simulink model "malt_test_angle"  (R2022a)
settings: Solver=FixedStepAuto  StartTime=0.0  StopTime=50  FixedStep=framePeriod_s  RelTol=1e-3
undefined symbols (not defined in the file): Aircraft, DiscIntNeverNeededParam, framePeriod_s
libraries: simulink x29, slpidlib x8, simulink_extras x3
(part 2 of 2)

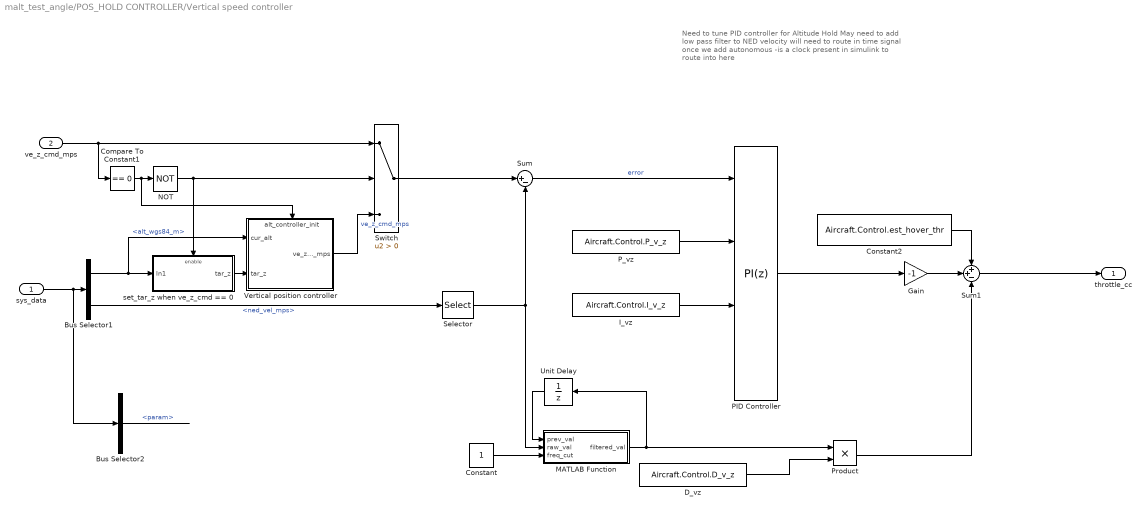
== system malt_test_angle/POS_HOLD CONTROLLER/Vertical speed controller ==
  note: Need to tune PID controller for Altitude Hold
      | May need to add low pass filter to NED velocity
      | will need to route in time signal once we add autonomous
      | -is a clock present in simulink to route into here
  sys_data : Inport
  ve_z_cmd_mps : Inport  Port=2
  Bus Selector1 : BusSelector  OutputSignals=Sensor Data.ext_gnss1.alt_wgs84_m,Sensor Data.ext_gnss1.ned_vel_mps
  Bus Selector2 : BusSelector  OutputSignals=Telemetry Data.param
  Compare To Constant1 : simulink/Logic and Bit Operations/Compare To Constant  relop===  const=0  OutDataTypeStr=boolean
  Constant : Constant
  Constant2 : Constant  Value=Aircraft.Control.est_hover_thr  OutDataTypeStr=single
  D_vz : Constant  Value=Aircraft.Control.D_v_z  OutDataTypeStr=single
  Gain : Gain  Gain=-1
  I_vz : Constant  Value=Aircraft.Control.I_v_z  OutDataTypeStr=single
  MATLAB Function : MATLAB Function  TreatAsAtomicUnit=on
  NOT : Logic  Operator=NOT  IconShape=distinctive  AllPortsSameDT=off  OutDataTypeStr=boolean
  PID Controller : slpidlib/PID Controller  Controller=PI  Form=Parallel  TimeDomain=Discrete-time  UseExternalTs=off  SampleTime=framePeriod_s  IntegratorMethod=Forward Euler  FilterMethod=Forward Euler  ControllerParametersSource=external  P=0  I=0  UseKiTs=off  D=0  N=100  UseFilter=off  TunerSelectOption=Frequency Response Based  InitialConditionSource=internal  InitialConditionForIntegrator=0  InitialConditionForFilter=0  DifferentiatorICPrevScaledInput=0  ExternalReset=either  TrackingMode=off  Kt=1  LimitOutput=on  SatLimitsSource=internal  UpperSaturationLimit=inf  LowerSaturationLimit=-inf  LinearizeAsGain=on  AntiWindupMode=clamping  Kb=1  POutMin=[]  POutMax=[]  IOutMin=[]  IOutMax=[]  DOutMin=[]  DOutMax=[]  NOutMin=[]  NOutMax=[]  SumOutMin=[]  SumOutMax=[]  SaturationOutMin=[]  SaturationOutMax=[]  PParamMin=[]  PParamMax=[]  IParamMin=[]  IParamMax=[]  DParamMin=[]  DParamMax=[]  NParamMin=[]  NParamMax=[]  KbParamMin=[]  KbParamMax=[]  KtParamMin=[]  KtParamMax=[]  KbOutMin=[]  KbOutMax=[]  KtOutMin=[]  KtOutMax=[]  IntegratorOutMin=[]  IntegratorOutMax=[]  FilterOutMin=[]  FilterOutMax=[]  SumI1OutMin=[]  SumI1OutMax=[]  SumI2OutMin=[]  SumI2OutMax=[]  SumI3OutMin=[]  SumI3OutMax=[]  SumI4OutMin=[]  SumI4OutMax=[]  SumDOutMin=[]  SumDOutMax=[]  DifferentiatorOutMin=[]  DifferentiatorOutMax=[]  FilterDiffOutCoefMin=[]  FilterDiffOutCoefMax=[]  ReciprocalOutMin=[]  ReciprocalOutMax=[]  SumDenOutMin=[]  SumDenOutMax=[]  SumNumOutMin=[]  SumNumOutMax=[]  DivideOutMin=[]  DivideOutMax=[]  UdiffTsProdOutMin=[]  UdiffTsProdOutMax=[]  NTsProdOutMin=[]  NTsProdOutMax=[]  UintegralTsProdOutMin=[]  UintegralTsProdOutMax=[]  UngainTsProdOutMin=[]  UngainTsProdOutMax=[]  IntegratorContinuousStateAttributes=''  IntegratorStateMustResolveToSignalObject=off  IntegratorRTWStateStorageClass=Auto  FilterContinuousStateAttributes=''  FilterStateMustResolveToSignalObject=off  FilterRTWStateStorageClass=Auto  ParallelPVariant=ExternalParameters  IdealPVariant=Disabled  IVariant=ExternalParameters  DVariant=Disabled  IntegratorVariant=Discrete  SatVariant=Enabled  AWVariant=DiscClampingParallel  PCopyVariant=Disabled  TRVariant=Disabled  FdbkBlocksVariant=Forward  IdealPFdbkVariant=Disabled  SatFdbkVariant=Disabled  DerivativeFilterVariant=Disabled  NVariant=Disabled  NCopyVariant=Disabled_SignalSpec  FilterICVariant=Disabled  IntegratorICVariant=InternalICs  ExternalResetVariant=ExternalReset  TRSumVariant=Passthrough  SumFdbkVariant=Disabled  SumVariant=Sum_PI  TsampFilterVariant=InternalTs  TsampNgainVariant=Passthrough  TsampIntegralVariant=Passthrough  ExternalSaturationOutDataTypeStr=Inherit: Same as second input  aMode=0
  P_vz : Constant  Value=Aircraft.Control.P_v_z  OutDataTypeStr=single
  Product : Product
  Selector : Selector  InputPortWidth=3  IndexOptions=Index vector (dialog)  Indices=[3]  OutputSizes=1
  Sum : Sum  Inputs=|+-
  Sum1 : Sum  Inputs=++-
  Switch : Switch  Criteria=u2 > Threshold  SaturateOnIntegerOverflow=off  InputSameDT=off
  Unit Delay : UnitDelay  SampleTime=-1  HasFrameUpgradeWarning=on
  Vertical position controller : Subsystem
      settings: PortSchema="{\"entries\":[{\"content\":{\"sides\":[{\"content\":{\"connectorIds\":[\"In1\",\"In2\"]},\"type\":\"ConnectorPlacement.EquallySpacedRectSide\",\"uuid\":\"4db66816-7259-4f9c-97dc-3e2ef8fc1f9a\"},{\"content\":{\"connectorIds\":[\"Out1\"],\"side\":\"RIGHT\"},\"type\":\"ConnectorPlacement.EquallySpacedRectSide\",\"uuid\":\"8b35fa77-d974-4b31-bf6a-1bec360e39d1\"},{\"content\":{\"connectorIds\":[\"In3\"],\"side\":\"TOP\"},\"type\":\"ConnectorPlacement.EquallySpacedRectSide\",\"uuid\":\"3ae99705-2896-4d33-823c-501dd4ab52dc\"}]},\"type\":\"ConnectorPlacement.EquallySpacedConnector\",\"uuid\":\"6b05b274-635e-41e6-a26b-037c1baff98b\"}],\"packageUris\":[\"http://schema.mathworks.com/mf0/Connector/R2020b\"],\"version\":\"1.0\"}"
  set_tar_z when ve_z_cmd == 0 : Subsystem  TreatAsAtomicUnit=on
  throttle_cc : Outport
  wires:
  Sum/1 -> PID Controller/1  "error"
  I_vz/1 -> PID Controller/3
  P_vz/1 -> PID Controller/2
  PID Controller/1 -> Gain/1
  Bus Selector1/2 -> Selector/1  "<ned_vel_mps>"
  sys_data/1 -> Bus Selector2/1, Bus Selector1/1
  Sum1/1 -> throttle_cc/1
  Bus Selector2/1 -> ?  "<param>"
  Unit Delay/1 -> MATLAB Function/1(prev_val)
  MATLAB Function/1(filtered_val) -> Product/1, Unit Delay/1
  Selector/1 -> Sum/2, MATLAB Function/2(raw_val)
  Constant/1 -> MATLAB Function/3(freq_cut)
  D_vz/1 -> Product/2
  Constant2/1 -> Sum1/1
  Gain/1 -> Sum1/2
  Product/1 -> Sum1/3
  ve_z_cmd_mps/1 -> Compare To Constant1/1, Switch/1
  Compare To Constant1/1 -> Vertical position controller/3(alt_controller_init), NOT/1
  Bus Selector1/1 -> Vertical position controller/1(cur_alt), set_tar_z when ve_z_cmd == 0/1(In1)  "<alt_wgs84_m>"
  NOT/1 -> Switch/2, set_tar_z when ve_z_cmd == 0/Enable
  Switch/1 -> Sum/1
  set_tar_z when ve_z_cmd == 0/1(tar_z) -> Vertical position controller/2(tar_z)
  Vertical position controller/1(ve_z_cmd_mps) -> Switch/3  "ve_z_cmd_mps"

== system malt_test_angle/Stab_input_conversion/remap from min_spin to max ==
  raw_in : Inport
  Constant4 : Constant  Value=0  OutDataTypeStr=single
  Constant5 : Constant  Value=Aircraft.Control.motor_spin_min  OutDataTypeStr=single
  Constant6 : Constant  OutDataTypeStr=single
  Constant7 : Constant  OutDataTypeStr=single
  remap1 : MATLAB Function  TreatAsAtomicUnit=on
  norm_out : Outport
  wires:
  Constant6/1 -> remap1/5(out_max)
  Constant5/1 -> remap1/4(out_min)
  remap1/1(norm_out) -> norm_out/1
  Constant4/1 -> remap1/2(in_min)
  Constant7/1 -> remap1/3(in_max)
  raw_in/1 -> remap1/1(raw_in)

== system malt_test_angle/Stab_input_conversion1/Throttle Mapper ==
  Throttle : Inport
  Compare To Constant : simulink/Logic and Bit Operations/Compare To Constant  relop=<  const=0  OutDataTypeStr=boolean
  Compare To Constant1 : simulink/Logic and Bit Operations/Compare To Constant  relop=>=  const=0  OutDataTypeStr=boolean
  Constant : Constant  Value=Aircraft.Control.v_z_down_max  OutDataTypeStr=single
  Constant1 : Constant  Value=Aircraft.Control.v_z_up_max  OutDataTypeStr=single
  Double : Constant  Value=2  OutDataTypeStr=single
  Gain : Gain  Gain=-1
  Normalize at Zero : Constant  Value=0.5  OutDataTypeStr=single
  Product : Product  Inputs=3
  Product1 : Product  Inputs=3
  Sum : Sum  Inputs=|+-
  Sum1 : Sum
  v_z_cmd (-1 to 1) : Product
  Relative Velocity : Outport
  wires:
  Throttle/1 -> Sum/1
  Normalize at Zero/1 -> Sum/2
  Double/1 -> v_z_cmd (-1 to 1)/2
  Sum/1 -> v_z_cmd (-1 to 1)/1
  Sum1/1 -> Gain/1
  v_z_cmd (-1 to 1)/1 -> Product1/2, Compare To Constant1/1, Compare To Constant/1, Product/3
  Constant1/1 -> Product1/3
  Compare To Constant1/1 -> Product1/1
  Product/1 -> Sum1/1
  Product1/1 -> Sum1/2
  Constant/1 -> Product/1
  Compare To Constant/1 -> Product/2
  Gain/1 -> Relative Velocity/1

== system malt_test_angle/Stab_input_conversion1/pitch_norm_deadband ==
  raw_sbus_in : Inport
  deadband : Inport  Port=2
  Constant : Constant  Value=0  OutDataTypeStr=single
  Constant1 : Constant  Value=0  OutDataTypeStr=single
  Constant2 : Constant  OutDataTypeStr=single
  Constant3 : Constant  OutDataTypeStr=single
  remap_with_deadband : MATLAB Function  TreatAsAtomicUnit=on
  normalized_out : Outport
  wires:
  deadband/1 -> remap_with_deadband/6(deadband)
  Constant2/1 -> remap_with_deadband/5(out_max)
  Constant1/1 -> remap_with_deadband/4(out_min)
  Constant3/1 -> remap_with_deadband/3(in_max)
  Constant/1 -> remap_with_deadband/2(in_min)
  remap_with_deadband/1(norm_out) -> normalized_out/1
  raw_sbus_in/1 -> remap_with_deadband/1(raw_in)

== system malt_test_angle/cmd to raw pwm1/motor_PWM_denormalize ==
  normalized_input : Inport
  Constant : Constant  Value=0  OutDataTypeStr=single
  Constant1 : Constant  Value=1100  OutDataTypeStr=single
  Constant2 : Constant  Value=1950  OutDataTypeStr=single
  Constant3 : Constant  OutDataTypeStr=single
  remap : MATLAB Function  TreatAsAtomicUnit=on
  raw_output : Outport
  wires:
  Constant2/1 -> remap/5(out_max)
  Constant1/1 -> remap/4(out_min)
  Constant3/1 -> remap/3(in_max)
  Constant/1 -> remap/2(in_min)
  remap/1(raw_out) -> raw_output/1
  normalized_input/1 -> remap/1(norm_in)

== system malt_test_angle/command selection/e_stop_norm ==
  raw_sbus_in : Inport
  Constant : Constant  Value=172  OutDataTypeStr=single
  Constant1 : Constant  Value=-1  OutDataTypeStr=single
  Constant2 : Constant  OutDataTypeStr=single
  Constant3 : Constant  Value=1811  OutDataTypeStr=single
  remap : MATLAB Function  TreatAsAtomicUnit=on
  normalized_out : Outport
  wires:
  Constant2/1 -> remap/5(out_max)
  Constant1/1 -> remap/4(out_min)
  Constant3/1 -> remap/3(in_max)
  Constant/1 -> remap/2(in_min)
  remap/1(norm_out) -> normalized_out/1
  raw_sbus_in/1 -> remap/1(raw_in)

== system malt_test_angle/command selection/mode_norm ==
  raw_sbus_in : Inport
  Constant : Constant  Value=172  OutDataTypeStr=single
  Constant1 : Constant  Value=0  OutDataTypeStr=single
  Constant2 : Constant  Value=2  OutDataTypeStr=single
  Constant3 : Constant  Value=1811  OutDataTypeStr=single
  remap : MATLAB Function  TreatAsAtomicUnit=on
  normalized_out : Outport
  wires:
  raw_sbus_in/1 -> remap/1(raw_in)
  remap/1(norm_out) -> normalized_out/1
  Constant/1 -> remap/2(in_min)
  Constant3/1 -> remap/3(in_max)
  Constant1/1 -> remap/4(out_min)
  Constant2/1 -> remap/5(out_max)

== system malt_test_angle/command selection/pitch_norm_deadband ==
  raw_sbus_in : Inport
  deadband : Inport  Port=2
  Constant : Constant  Value=172  OutDataTypeStr=single
  Constant1 : Constant  Value=-1  OutDataTypeStr=single
  Constant2 : Constant  OutDataTypeStr=single
  Constant3 : Constant  Value=1811  OutDataTypeStr=single
  remap_with_deadband : MATLAB Function  TreatAsAtomicUnit=on
  normalized_out : Outport
  wires:
  deadband/1 -> remap_with_deadband/6(deadband)
  Constant2/1 -> remap_with_deadband/5(out_max)
  Constant1/1 -> remap_with_deadband/4(out_min)
  Constant3/1 -> remap_with_deadband/3(in_max)
  Constant/1 -> remap_with_deadband/2(in_min)
  remap_with_deadband/1(norm_out) -> normalized_out/1
  raw_sbus_in/1 -> remap_with_deadband/1(raw_in)

== system malt_test_angle/command selection/roll_norm_deadband ==
  raw_sbus_in : Inport
  deadband : Inport  Port=2
  Constant : Constant  Value=172  OutDataTypeStr=single
  Constant1 : Constant  Value=-1  OutDataTypeStr=single
  Constant2 : Constant  OutDataTypeStr=single
  Constant3 : Constant  Value=1811  OutDataTypeStr=single
  remap_with_deadband : MATLAB Function  TreatAsAtomicUnit=on
  normalized_out : Outport
  wires:
  deadband/1 -> remap_with_deadband/6(deadband)
  Constant2/1 -> remap_with_deadband/5(out_max)
  Constant1/1 -> remap_with_deadband/4(out_min)
  Constant3/1 -> remap_with_deadband/3(in_max)
  Constant/1 -> remap_with_deadband/2(in_min)
  remap_with_deadband/1(norm_out) -> normalized_out/1
  raw_sbus_in/1 -> remap_with_deadband/1(raw_in)

== system malt_test_angle/command selection/throttle_norm ==
  raw_sbus_in : Inport
  Constant : Constant  Value=172  OutDataTypeStr=single
  Constant1 : Constant  Value=0  OutDataTypeStr=single
  Constant2 : Constant  OutDataTypeStr=single
  Constant3 : Constant  Value=1811  OutDataTypeStr=single
  remap : MATLAB Function  TreatAsAtomicUnit=on
  normalized_out : Outport
  wires:
  raw_sbus_in/1 -> remap/1(raw_in)
  remap/1(norm_out) -> normalized_out/1
  Constant/1 -> remap/2(in_min)
  Constant3/1 -> remap/3(in_max)
  Constant1/1 -> remap/4(out_min)
  Constant2/1 -> remap/5(out_max)

== system malt_test_angle/command selection/yaw_norm_deadband ==
  raw_sbus_in : Inport
  deadband : Inport  Port=2
  Constant : Constant  Value=172  OutDataTypeStr=single
  Constant1 : Constant  Value=-1  OutDataTypeStr=single
  Constant2 : Constant  OutDataTypeStr=single
  Constant3 : Constant  Value=1811  OutDataTypeStr=single
  remap_with_deadband : MATLAB Function  TreatAsAtomicUnit=on
  normalized_out : Outport
  wires:
  raw_sbus_in/1 -> remap_with_deadband/1(raw_in)
  remap_with_deadband/1(norm_out) -> normalized_out/1
  Constant/1 -> remap_with_deadband/2(in_min)
  Constant3/1 -> remap_with_deadband/3(in_max)
  Constant1/1 -> remap_with_deadband/4(out_min)
  Constant2/1 -> remap_with_deadband/5(out_max)
  deadband/1 -> remap_with_deadband/6(deadband)

== system malt_test_angle/determine arm and mode selection/Failsafe_management ==
  note: - radio failsafe
  In Bus Element1 : Inport  PortName=failsafe  Element=failsafe
  manual_mode : Inport  Port=2
  motor_state : Inport  Port=3
  NOT : Logic  Operator=NOT  IconShape=distinctive  AllPortsSameDT=off  OutDataTypeStr=boolean
  Radio failsafe : Subsystem
  radio_failsafe_enabled : Outport
  wires:
  Radio failsafe/1(radio_failsafe_enabled) -> radio_failsafe_enabled/1
  manual_mode/1 -> [manual_mode], Radio failsafe/2(manual_mode)
  motor_state/1 -> Radio failsafe/3(motor_state)
  In Bus Element1/1 -> NOT/1
  NOT/1 -> Radio failsafe/1(failsafe)

== system malt_test_angle/determine arm and mode selection/Subsystem ==
  <e_stop> : Inport
  Abs1 : Abs  SaturateOnIntegerOverflow=off
  Compare To Constant : simulink/Logic and Bit Operations/Compare To Constant  relop=>=  const=0.98  OutDataTypeStr=boolean
  e_stop counter : Subsystem
  e_stop_filtered : Outport
  wires:
  Compare To Constant/1 -> e_stop counter/Enable
  Abs1/1 -> Compare To Constant/1
  <e_stop>/1 -> e_stop counter/1(motor_e_stop_raw), Abs1/1
  e_stop counter/1(e_stop_filtered) -> e_stop_filtered/1

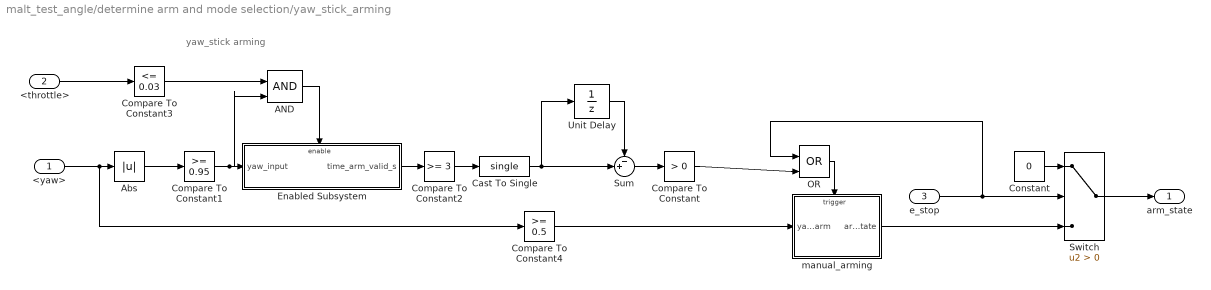
== system malt_test_angle/determine arm and mode selection/yaw_stick_arming ==
  note: yaw_stick arming
  <yaw> : Inport
  <throttle> : Inport  Port=2
  e_stop : Inport  Port=3
  AND : Logic  IconShape=distinctive  AllPortsSameDT=off  OutDataTypeStr=boolean
  Abs : Abs  SaturateOnIntegerOverflow=off
  Cast To Single : DataTypeConversion  OutDataTypeStr=single  SaturateOnIntegerOverflow=off  RndMeth=Floor
  Compare To Constant : simulink/Logic and Bit Operations/Compare To Constant  relop=>  const=0  OutDataTypeStr=boolean
  Compare To Constant1 : simulink/Logic and Bit Operations/Compare To Constant  relop=>=  const=0.95  OutDataTypeStr=boolean
  Compare To Constant2 : simulink/Logic and Bit Operations/Compare To Constant  relop=>=  const=3  OutDataTypeStr=boolean
  Compare To Constant3 : simulink/Logic and Bit Operations/Compare To Constant  relop=<=  const=0.03  OutDataTypeStr=boolean
  Compare To Constant4 : simulink/Logic and Bit Operations/Compare To Constant  relop=>=  const=0.5  OutDataTypeStr=boolean
  Constant : Constant  Value=0  OutDataTypeStr=boolean  LockScale=on
  Enabled Subsystem : Subsystem  TreatAsAtomicUnit=on
  OR : Logic  Operator=OR  IconShape=distinctive  AllPortsSameDT=off  OutDataTypeStr=boolean
  Sum : Sum  Inputs=-+|
  Switch : Switch  Criteria=u2 > Threshold  SaturateOnIntegerOverflow=off  InputSameDT=off
  Unit Delay : UnitDelay  SampleTime=-1  HasFrameUpgradeWarning=on
  manual_arming : Subsystem
  arm_state : Outport
  wires:
  Enabled Subsystem/1(time_arm_valid_s) -> Compare To Constant2/1
  Abs/1 -> Compare To Constant1/1
  Compare To Constant1/1 -> AND/2, Enabled Subsystem/1(yaw_input)
  Compare To Constant4/1 -> manual_arming/1(yaw_arm)
  AND/1 -> Enabled Subsystem/Enable
  <yaw>/1 -> Compare To Constant4/1, Abs/1
  <throttle>/1 -> Compare To Constant3/1
  Compare To Constant3/1 -> AND/1
  Constant/1 -> Switch/1
  manual_arming/1(arm_state) -> Switch/3
  Switch/1 -> arm_state/1
  e_stop/1 -> OR/1, Switch/2
  OR/1 -> manual_arming/Trigger
  Compare To Constant2/1 -> Cast To Single/1
  Sum/1 -> Compare To Constant/1
  Unit Delay/1 -> Sum/1
  Cast To Single/1 -> Unit Delay/1, Sum/2
  Compare To Constant/1 -> OR/2

== system malt_test_angle/ANGLE CONTROLLER1/Pitch Controller/Pitch_D_DLPF ==
  raw_val : Inport
  freq_cut : Inport  Port=2
  MATLAB Function : MATLAB Function  TreatAsAtomicUnit=on
  Unit Delay : UnitDelay  SampleTime=-1  HasFrameUpgradeWarning=on
  filtered_val : Outport
  wires:
  MATLAB Function/1(filtered_val) -> filtered_val/1, Unit Delay/1
  raw_val/1 -> MATLAB Function/2(raw_val)
  Unit Delay/1 -> MATLAB Function/1(prev_val)
  freq_cut/1 -> MATLAB Function/3(freq_cut)

== system malt_test_angle/ANGLE CONTROLLER1/Roll Controller/roll_D_DLPF ==
  raw_val : Inport
  freq_cut : Inport  Port=2
  MATLAB Function : MATLAB Function  TreatAsAtomicUnit=on
  Unit Delay : UnitDelay  SampleTime=-1  HasFrameUpgradeWarning=on
  filtered_val : Outport
  wires:
  freq_cut/1 -> MATLAB Function/3(freq_cut)
  MATLAB Function/1(filtered_val) -> filtered_val/1, Unit Delay/1
  Unit Delay/1 -> MATLAB Function/1(prev_val)
  raw_val/1 -> MATLAB Function/2(raw_val)

== system malt_test_angle/ANGLE CONTROLLER1/Yaw Rate Controller/heading_error ==
  heading_cmd_rad : Inport
  heading_rad : Inport  Port=2
  Abs : Abs  SaturateOnIntegerOverflow=off
  Compare To Constant : simulink/Logic and Bit Operations/Compare To Constant  relop=>  const=pi  OutDataTypeStr=boolean
  Constant : Constant  Value=2*pi  OutDataTypeStr=single
  Product : Product
  Sign : Signum
  Subtract : Sum  Inputs=+-
  Subtract1 : Sum  Inputs=+-
  Switch : Switch  Criteria=u2 > Threshold  SaturateOnIntegerOverflow=off  InputSameDT=off
  heading_error_rad : Outport
  wires:
  heading_cmd_rad/1 -> Subtract/1
  heading_rad/1 -> Subtract/2
  Subtract/1 -> Abs/1, Switch/3, Subtract1/1, Sign/1
  Compare To Constant/1 -> Switch/2
  Subtract1/1 -> Switch/1
  Switch/1 -> heading_error_rad/1
  Abs/1 -> Compare To Constant/1
  Sign/1 -> Product/1
  Product/1 -> Subtract1/2
  Constant/1 -> Product/2

== system malt_test_angle/ANGLE CONTROLLER1/Yaw Rate Controller/set_tar_heading when heading_rate_cmd == 0 ==
  heading_rad : Inport
  Enable : EnablePort
  target_heading_rad : Outport
  wires:
  heading_rad/1 -> target_heading_rad/1

== system malt_test_angle/ANGLE CONTROLLER1/Yaw Rate Controller/yaw_D_DLPF ==
  raw_val : Inport
  freq_cut : Inport  Port=2
  MATLAB Function : MATLAB Function  TreatAsAtomicUnit=on
  Unit Delay : UnitDelay  SampleTime=-1  HasFrameUpgradeWarning=on
  filtered_val : Outport
  wires:
  Unit Delay/1 -> MATLAB Function/1(prev_val)
  raw_val/1 -> MATLAB Function/2(raw_val)
  MATLAB Function/1(filtered_val) -> filtered_val/1, Unit Delay/1
  freq_cut/1 -> MATLAB Function/3(freq_cut)

== system malt_test_angle/POS_HOLD CONTROLLER/Horizontal speed controller/2D rotation from NED_xy to body_xy ==
  <heading_rad> : Inport
  Cos : Trigonometry  Operator=cos  OutputSignalType=real
  Gain : Gain  Gain=-1
  Mux : Mux
  Reshape : Reshape  OutputDimensionality=Customize  OutputDimensions=[2,2]
  Sin : Trigonometry  OutputSignalType=real
  2D_rot : Outport
  wires:
  <heading_rad>/1 -> Sin/1, Cos/1
  Mux/1 -> Reshape/1
  Sin/1 -> Mux/3, Gain/1
  Cos/1 -> Mux/1, Mux/4
  Reshape/1 -> 2D_rot/1
  Gain/1 -> Mux/2

== system malt_test_angle/POS_HOLD CONTROLLER/Horizontal speed controller/Subsystem ==
  vb_x cmd : Inport
  vb_x : Inport  Port=2
  pos_hold_p : Inport  Port=3
  pos_hold_I : Inport  Port=4
  pos_hold_D : Inport  Port=5
  pos_hold_init : Inport  Port=6
  Gain : Gain  Gain=-1
  Gain Selector : Subsystem  Commented=through
  Gain Selector1 : Subsystem  Commented=through
  Gain Selector2 : Subsystem  Commented=through
  Pitch angle controller : slpidlib/PID Controller  Controller=PID  Form=Parallel  TimeDomain=Discrete-time  UseExternalTs=off  SampleTime=framePeriod_s  IntegratorMethod=Forward Euler  FilterMethod=Forward Euler  ControllerParametersSource=external  P=0.335  I=0.005  UseKiTs=off  D=0  N=100  UseFilter=off  TunerSelectOption=Transfer Function Based (PID Tuner App)  InitialConditionSource=internal  InitialConditionForIntegrator=0  InitialConditionForFilter=0  DifferentiatorICPrevScaledInput=0  ExternalReset=rising  TrackingMode=off  Kt=1  LimitOutput=on  SatLimitsSource=internal  UpperSaturationLimit=inf  LowerSaturationLimit=-inf  LinearizeAsGain=off  AntiWindupMode=clamping  Kb=1  POutMin=[]  POutMax=[]  IOutMin=[]  IOutMax=[]  DOutMin=[]  DOutMax=[]  NOutMin=[]  NOutMax=[]  SumOutMin=[]  SumOutMax=[]  SaturationOutMin=[]  SaturationOutMax=[]  PParamMin=[]  PParamMax=[]  IParamMin=[]  IParamMax=[]  DParamMin=[]  DParamMax=[]  NParamMin=[]  NParamMax=[]  KbParamMin=[]  KbParamMax=[]  KtParamMin=[]  KtParamMax=[]  KbOutMin=[]  KbOutMax=[]  KtOutMin=[]  KtOutMax=[]  IntegratorOutMin=[]  IntegratorOutMax=[]  FilterOutMin=[]  FilterOutMax=[]  SumI1OutMin=[]  SumI1OutMax=[]  SumI2OutMin=[]  SumI2OutMax=[]  SumI3OutMin=[]  SumI3OutMax=[]  SumI4OutMin=[]  SumI4OutMax=[]  SumDOutMin=[]  SumDOutMax=[]  DifferentiatorOutMin=[]  DifferentiatorOutMax=[]  FilterDiffOutCoefMin=[]  FilterDiffOutCoefMax=[]  ReciprocalOutMin=[]  ReciprocalOutMax=[]  SumDenOutMin=[]  SumDenOutMax=[]  SumNumOutMin=[]  SumNumOutMax=[]  DivideOutMin=[]  DivideOutMax=[]  UdiffTsProdOutMin=[]  UdiffTsProdOutMax=[]  NTsProdOutMin=[]  NTsProdOutMax=[]  UintegralTsProdOutMin=[]  UintegralTsProdOutMax=[]  UngainTsProdOutMin=[]  UngainTsProdOutMax=[]  IntegratorContinuousStateAttributes=''  IntegratorStateMustResolveToSignalObject=off  IntegratorRTWStateStorageClass=Auto  FilterContinuousStateAttributes=''  FilterStateMustResolveToSignalObject=off  FilterRTWStateStorageClass=Auto  ParallelPVariant=ExternalParameters  IdealPVariant=Disabled  IVariant=ExternalParameters  DVariant=ExternalParameters  IntegratorVariant=Discrete  SatVariant=Enabled  AWVariant=DiscClampingParallel  PCopyVariant=Disabled  TRVariant=Disabled  FdbkBlocksVariant=Forward  IdealPFdbkVariant=Disabled  SatFdbkVariant=Disabled  DerivativeFilterVariant=Differentiator  NVariant=Passthrough  NCopyVariant=Disabled_SignalSpec  FilterICVariant=InternalICsDifferentiator  IntegratorICVariant=InternalICs  ExternalResetVariant=ExternalReset  TRSumVariant=Passthrough  SumFdbkVariant=Disabled  SumVariant=Sum_PID  TsampFilterVariant=InternalTs  TsampNgainVariant=Passthrough  TsampIntegralVariant=Passthrough  ExternalSaturationOutDataTypeStr=Inherit: Same as second input  aMode=0
  Saturation : Saturate  UpperLimit=Aircraft.Control.pitch_angle_lim  LowerLimit=-Aircraft.Control.pitch_angle_lim  LinearizeAsGain=off
  Sum : Sum  Inputs=|+-
  pitch_cmd_rad : Outport
  wires:
  vb_x/1 -> Sum/2
  Sum/1 -> Pitch angle controller/1
  vb_x cmd/1 -> Sum/1
  Saturation/1 -> Gain/1
  Pitch angle controller/1 -> Saturation/1
  Gain/1 -> pitch_cmd_rad/1
  pos_hold_I/1 -> Gain Selector1/1(param)
  pos_hold_p/1 -> Gain Selector/1(param)
  Gain Selector/1(gain) -> Pitch angle controller/2
  Gain Selector1/1(gain) -> Pitch angle controller/3  "I_gain"
  Gain Selector2/1(gain) -> Pitch angle controller/4  "I_gain"
  pos_hold_D/1 -> Gain Selector2/1(param)
  pos_hold_init/1 -> Pitch angle controller/5

== system malt_test_angle/POS_HOLD CONTROLLER/Horizontal speed controller/Subsystem1 ==
  vb_y : Inport
  vb_y cmd : Inport  Port=2
  pos_hold_p : Inport  Port=3
  pos_hold_I : Inport  Port=4
  pos_hold_D : Inport  Port=5
  pos_hold_init : Inport  Port=6
  Gain Selector : Subsystem  Commented=through
  Gain Selector1 : Subsystem  Commented=through
  Gain Selector2 : Subsystem  Commented=through
  Roll angle controller : slpidlib/PID Controller  Controller=PID  Form=Parallel  TimeDomain=Discrete-time  UseExternalTs=off  SampleTime=framePeriod_s  IntegratorMethod=Forward Euler  FilterMethod=Forward Euler  ControllerParametersSource=external  P=0.335  I=0.005  UseKiTs=off  D=0  N=100  UseFilter=off  TunerSelectOption=Transfer Function Based (PID Tuner App)  InitialConditionSource=internal  InitialConditionForIntegrator=0  InitialConditionForFilter=0  DifferentiatorICPrevScaledInput=0  ExternalReset=rising  TrackingMode=off  Kt=1  LimitOutput=on  SatLimitsSource=internal  UpperSaturationLimit=inf  LowerSaturationLimit=-inf  LinearizeAsGain=off  AntiWindupMode=clamping  Kb=1  POutMin=[]  POutMax=[]  IOutMin=[]  IOutMax=[]  DOutMin=[]  DOutMax=[]  NOutMin=[]  NOutMax=[]  SumOutMin=[]  SumOutMax=[]  SaturationOutMin=[]  SaturationOutMax=[]  PParamMin=[]  PParamMax=[]  IParamMin=[]  IParamMax=[]  DParamMin=[]  DParamMax=[]  NParamMin=[]  NParamMax=[]  KbParamMin=[]  KbParamMax=[]  KtParamMin=[]  KtParamMax=[]  KbOutMin=[]  KbOutMax=[]  KtOutMin=[]  KtOutMax=[]  IntegratorOutMin=[]  IntegratorOutMax=[]  FilterOutMin=[]  FilterOutMax=[]  SumI1OutMin=[]  SumI1OutMax=[]  SumI2OutMin=[]  SumI2OutMax=[]  SumI3OutMin=[]  SumI3OutMax=[]  SumI4OutMin=[]  SumI4OutMax=[]  SumDOutMin=[]  SumDOutMax=[]  DifferentiatorOutMin=[]  DifferentiatorOutMax=[]  FilterDiffOutCoefMin=[]  FilterDiffOutCoefMax=[]  ReciprocalOutMin=[]  ReciprocalOutMax=[]  SumDenOutMin=[]  SumDenOutMax=[]  SumNumOutMin=[]  SumNumOutMax=[]  DivideOutMin=[]  DivideOutMax=[]  UdiffTsProdOutMin=[]  UdiffTsProdOutMax=[]  NTsProdOutMin=[]  NTsProdOutMax=[]  UintegralTsProdOutMin=[]  UintegralTsProdOutMax=[]  UngainTsProdOutMin=[]  UngainTsProdOutMax=[]  IntegratorContinuousStateAttributes=''  IntegratorStateMustResolveToSignalObject=off  IntegratorRTWStateStorageClass=Auto  FilterContinuousStateAttributes=''  FilterStateMustResolveToSignalObject=off  FilterRTWStateStorageClass=Auto  ParallelPVariant=ExternalParameters  IdealPVariant=Disabled  IVariant=ExternalParameters  DVariant=ExternalParameters  IntegratorVariant=Discrete  SatVariant=Enabled  AWVariant=DiscClampingParallel  PCopyVariant=Disabled  TRVariant=Disabled  FdbkBlocksVariant=Forward  IdealPFdbkVariant=Disabled  SatFdbkVariant=Disabled  DerivativeFilterVariant=Differentiator  NVariant=Passthrough  NCopyVariant=Disabled_SignalSpec  FilterICVariant=InternalICsDifferentiator  IntegratorICVariant=InternalICs  ExternalResetVariant=ExternalReset  TRSumVariant=Passthrough  SumFdbkVariant=Disabled  SumVariant=Sum_PID  TsampFilterVariant=InternalTs  TsampNgainVariant=Passthrough  TsampIntegralVariant=Passthrough  ExternalSaturationOutDataTypeStr=Inherit: Same as second input  aMode=0
  Saturation : Saturate  UpperLimit=Aircraft.Control.pitch_angle_lim  LowerLimit=-Aircraft.Control.pitch_angle_lim  LinearizeAsGain=off
  Sum : Sum  Inputs=|+-
  roll_cmd_rad : Outport
  wires:
  vb_y/1 -> Sum/2
  Gain Selector1/1(gain) -> Roll angle controller/3
  Gain Selector2/1(gain) -> Roll angle controller/4
  Sum/1 -> Roll angle controller/1
  Gain Selector/1(gain) -> Roll angle controller/2
  Saturation/1 -> roll_cmd_rad/1
  Roll angle controller/1 -> Saturation/1
  vb_y cmd/1 -> Sum/1
  pos_hold_I/1 -> Gain Selector1/1(param)
  pos_hold_p/1 -> Gain Selector/1(param)
  pos_hold_D/1 -> Gain Selector2/1(param)
  pos_hold_init/1 -> Roll angle controller/5

== system malt_test_angle/POS_HOLD CONTROLLER/Vertical speed controller/Vertical position controller ==
  cur_alt : Inport
  tar_z : Inport  Port=2
  alt_controller_init : Inport  Port=3
  Altitude PID : slpidlib/PID Controller  Controller=PI  Form=Ideal  TimeDomain=Discrete-time  UseExternalTs=off  SampleTime=framePeriod_s  IntegratorMethod=Forward Euler  FilterMethod=Forward Euler  ControllerParametersSource=external  P=0  I=0  UseKiTs=off  D=0  N=100  UseFilter=off  TunerSelectOption=Frequency Response Based  ZeroCross=off  InitialConditionSource=internal  InitialConditionForIntegrator=0  InitialConditionForFilter=0  DifferentiatorICPrevScaledInput=0  ExternalReset=rising  TrackingMode=off  Kt=1  LimitOutput=on  SatLimitsSource=internal  UpperSaturationLimit=Aircraft.Control.v_z_up_max  LowerSaturationLimit=-Aircraft.Control.v_z_down_max  LinearizeAsGain=on  AntiWindupMode=clamping  Kb=1  POutMin=[]  POutMax=[]  IOutMin=[]  IOutMax=[]  DOutMin=[]  DOutMax=[]  NOutMin=[]  NOutMax=[]  SumOutMin=[]  SumOutMax=[]  SaturationOutMin=[]  SaturationOutMax=[]  PParamMin=[]  PParamMax=[]  IParamMin=[]  IParamMax=[]  DParamMin=[]  DParamMax=[]  NParamMin=[]  NParamMax=[]  KbParamMin=[]  KbParamMax=[]  KtParamMin=[]  KtParamMax=[]  KbOutMin=[]  KbOutMax=[]  KtOutMin=[]  KtOutMax=[]  IntegratorOutMin=[]  IntegratorOutMax=[]  FilterOutMin=[]  FilterOutMax=[]  SumI1OutMin=[]  SumI1OutMax=[]  SumI2OutMin=[]  SumI2OutMax=[]  SumI3OutMin=[]  SumI3OutMax=[]  SumI4OutMin=[]  SumI4OutMax=[]  SumDOutMin=[]  SumDOutMax=[]  DifferentiatorOutMin=[]  DifferentiatorOutMax=[]  FilterDiffOutCoefMin=[]  FilterDiffOutCoefMax=[]  ReciprocalOutMin=[]  ReciprocalOutMax=[]  SumDenOutMin=[]  SumDenOutMax=[]  SumNumOutMin=[]  SumNumOutMax=[]  DivideOutMin=[]  DivideOutMax=[]  UdiffTsProdOutMin=[]  UdiffTsProdOutMax=[]  NTsProdOutMin=[]  NTsProdOutMax=[]  UintegralTsProdOutMin=[]  UintegralTsProdOutMax=[]  UngainTsProdOutMin=[]  UngainTsProdOutMax=[]  IntegratorContinuousStateAttributes=''  IntegratorStateMustResolveToSignalObject=off  IntegratorRTWStateStorageClass=Auto  FilterContinuousStateAttributes=''  FilterStateMustResolveToSignalObject=off  FilterRTWStateStorageClass=Auto  ParallelPVariant=Passthrough  IdealPVariant=ExternalParameters  IVariant=ExternalParameters  DVariant=Disabled  IntegratorVariant=Discrete  SatVariant=Enabled  AWVariant=DiscClampingIdeal  PCopyVariant=ExternalParamsIdeal  TRVariant=Disabled  FdbkBlocksVariant=Forward  IdealPFdbkVariant=Disabled  SatFdbkVariant=Disabled  DerivativeFilterVariant=Disabled  NVariant=Disabled  NCopyVariant=Disabled_SignalSpec  FilterICVariant=Disabled  IntegratorICVariant=InternalICs  ExternalResetVariant=ExternalReset  TRSumVariant=Passthrough  SumFdbkVariant=Disabled  SumVariant=Sum_PI  TsampFilterVariant=InternalTs  TsampNgainVariant=Passthrough  TsampIntegralVariant=Passthrough  ExternalSaturationOutDataTypeStr=Inherit: Same as second input  aMode=0
  P_alt : Constant  Value=Aircraft.Control.P_alt  OutDataTypeStr=single
  P_alt1 : Constant  Value=Aircraft.Control.I_alt  OutDataTypeStr=single
  Sum3 : Sum  Inputs=|+-
  ve_z_cmd_mps : Outport
  wires:
  Altitude PID/1 -> ve_z_cmd_mps/1
  tar_z/1 -> Sum3/1  "target_z"
  cur_alt/1 -> Sum3/2
  P_alt1/1 -> Altitude PID/3
  Sum3/1 -> Altitude PID/1
  P_alt/1 -> Altitude PID/2
  alt_controller_init/1 -> Altitude PID/4

== system malt_test_angle/POS_HOLD CONTROLLER/Vertical speed controller/set_tar_z when ve_z_cmd == 0 ==
  In1 : Inport
  Enable : EnablePort
  tar_z : Outport
  wires:
  In1/1 -> tar_z/1

== system malt_test_angle/determine arm and mode selection/Failsafe_management/Radio failsafe ==
  note: Transition to RTL mode
  note: If radio_failsafe is triggered and current_mode is not auto, rtl, land nor motor_state disarmed then RTL mode is triggered
  failsafe : Inport
  manual_mode : Inport  Port=2
  motor_state : Inport  Port=3
  AND1 : Logic  Commented=on  IconShape=distinctive  AllPortsSameDT=off  OutDataTypeStr=boolean
  Compare To Constant : simulink/Logic and Bit Operations/Compare To Constant  Commented=on  relop=~=  const=3  OutDataTypeStr=boolean
  Compare To Constant1 : simulink/Logic and Bit Operations/Compare To Constant  Commented=on  relop=~=  const=4  OutDataTypeStr=boolean
  Compare To Constant2 : simulink/Logic and Bit Operations/Compare To Constant  Commented=on  relop=~=  const=5  OutDataTypeStr=boolean
  NOR : Logic  Commented=on  Operator=NOR  Inputs=4  IconShape=distinctive  AllPortsSameDT=off  OutDataTypeStr=boolean
  NOT : Logic  Commented=on  Operator=NOT  IconShape=distinctive  AllPortsSameDT=off  OutDataTypeStr=boolean
  NOT1 : Logic  Operator=NOT  IconShape=distinctive  AllPortsSameDT=off  OutDataTypeStr=boolean
  Subsystem : Subsystem
  radio_failsafe_enabled : Outport
  wires:
  manual_mode/1 -> Compare To Constant2/1, Compare To Constant1/1, Compare To Constant/1
  Compare To Constant/1 -> NOR/1
  Compare To Constant1/1 -> NOR/2
  Compare To Constant2/1 -> NOR/3
  motor_state/1 -> NOT/1
  NOT/1 -> NOR/4
  failsafe/1 -> Subsystem/1(<inceptor_health>)
  NOR/1 -> AND1/1
  Subsystem/1(inceptor_health_filtered) -> NOT1/1
  NOT1/1 -> radio_failsafe_enabled/1

== system malt_test_angle/determine arm and mode selection/Subsystem/e_stop counter ==
  note: This is to ensure e_stop event is not triggered unless e_stop command is sent for more than 0.3 s to prevent false trigger
  motor_e_stop_raw : Inport
  Enable : EnablePort  StatesWhenEnabling=reset
  Compare To Constant : simulink/Logic and Bit Operations/Compare To Constant  relop=>=  const=0.5  OutDataTypeStr=boolean
  Discrete-Time Integrator : DiscreteIntegrator  SampleTime=0.01  LimitOutput=on  UpperSaturationLimit=1  LowerSaturationLimit=0  ICPrevOutput=DiscIntNeverNeededParam  ICPrevScaledInput=DiscIntNeverNeededParam
  Gain : Gain  Gain=2
  e_stop_filtered : Outport
  wires:
  Compare To Constant/1 -> e_stop_filtered/1
  Discrete-Time Integrator/1 -> Compare To Constant/1
  Gain/1 -> Discrete-Time Integrator/1
  motor_e_stop_raw/1 -> Gain/1

== system malt_test_angle/determine arm and mode selection/yaw_stick_arming/Enabled Subsystem ==
  yaw_input : Inport
  Enable : EnablePort  StatesWhenEnabling=reset
  Cast : DataTypeConversion  OutDataTypeStr=int8  SaturateOnIntegerOverflow=off  RndMeth=Floor
  Discrete-Time Integrator : DiscreteIntegrator  IntegratorMethod=Integration: Trapezoidal  SampleTime=-1  OutDataTypeStr=single  UpperSaturationLimit=1  LowerSaturationLimit=0  ICPrevOutput=DiscIntNeverNeededParam  ICPrevScaledInput=DiscIntNeverNeededParam
  time_arm_valid_s : Outport
  wires:
  Discrete-Time Integrator/1 -> time_arm_valid_s/1
  Cast/1 -> Discrete-Time Integrator/1
  yaw_input/1 -> Cast/1

== system malt_test_angle/determine arm and mode selection/yaw_stick_arming/manual_arming ==
  yaw_arm : Inport
  Trigger : TriggerPort  VariantControl=(inherit)  PortDimensions=1
  arm_state : Outport
  wires:
  yaw_arm/1 -> arm_state/1

== system malt_test_angle/POS_HOLD CONTROLLER/Horizontal speed controller/Subsystem/Gain Selector ==
  param : Inport
  Constant : Constant  Value=Aircraft.Control.P_v_hor  OutDataTypeStr=single
  Constant1 : Constant  Value=Aircraft.Control.hardcode_values
  Switch : Switch  Criteria=u2 > Threshold  SaturateOnIntegerOverflow=off  InputSameDT=off
  gain : Outport
  wires:
  Constant/1 -> Switch/1
  Constant1/1 -> Switch/2
  param/1 -> Switch/3
  Switch/1 -> gain/1

== system malt_test_angle/POS_HOLD CONTROLLER/Horizontal speed controller/Subsystem/Gain Selector1 ==
  param : Inport
  Constant1 : Constant  Value=Aircraft.Control.hardcode_values
  Constant2 : Constant  Value=Aircraft.Control.I_v_hor  OutDataTypeStr=single
  Switch : Switch  Criteria=u2 > Threshold  SaturateOnIntegerOverflow=off  InputSameDT=off
  gain : Outport
  wires:
  Switch/1 -> gain/1
  param/1 -> Switch/3
  Constant1/1 -> Switch/2
  Constant2/1 -> Switch/1

== system malt_test_angle/POS_HOLD CONTROLLER/Horizontal speed controller/Subsystem/Gain Selector2 ==
  param : Inport
  Constant1 : Constant  Value=Aircraft.Control.hardcode_values
  Constant2 : Constant  Value=Aircraft.Control.D_v_hor  OutDataTypeStr=single
  Switch : Switch  Criteria=u2 > Threshold  SaturateOnIntegerOverflow=off  InputSameDT=off
  gain : Outport
  wires:
  Switch/1 -> gain/1
  param/1 -> Switch/3
  Constant1/1 -> Switch/2
  Constant2/1 -> Switch/1

== system malt_test_angle/POS_HOLD CONTROLLER/Horizontal speed controller/Subsystem1/Gain Selector ==
  param : Inport
  Constant : Constant  Value=Aircraft.Control.P_v_hor  OutDataTypeStr=single
  Constant1 : Constant  Value=Aircraft.Control.hardcode_values
  Switch : Switch  Criteria=u2 > Threshold  SaturateOnIntegerOverflow=off  InputSameDT=off
  gain : Outport
  wires:
  Constant/1 -> Switch/1
  Constant1/1 -> Switch/2
  param/1 -> Switch/3
  Switch/1 -> gain/1

== system malt_test_angle/POS_HOLD CONTROLLER/Horizontal speed controller/Subsystem1/Gain Selector1 ==
  param : Inport
  Constant1 : Constant  Value=Aircraft.Control.hardcode_values
  Constant2 : Constant  Value=Aircraft.Control.I_v_hor  OutDataTypeStr=single
  Switch : Switch  Criteria=u2 > Threshold  SaturateOnIntegerOverflow=off  InputSameDT=off
  gain : Outport
  wires:
  Switch/1 -> gain/1
  param/1 -> Switch/3
  Constant1/1 -> Switch/2
  Constant2/1 -> Switch/1

== system malt_test_angle/POS_HOLD CONTROLLER/Horizontal speed controller/Subsystem1/Gain Selector2 ==
  param : Inport
  Constant1 : Constant  Value=Aircraft.Control.hardcode_values
  Constant2 : Constant  Value=Aircraft.Control.D_v_hor  OutDataTypeStr=single
  Switch : Switch  Criteria=u2 > Threshold  SaturateOnIntegerOverflow=off  InputSameDT=off
  gain : Outport
  wires:
  Switch/1 -> gain/1
  param/1 -> Switch/3
  Constant1/1 -> Switch/2
  Constant2/1 -> Switch/1

== system malt_test_angle/determine arm and mode selection/Failsafe_management/Radio failsafe/Subsystem ==
  <inceptor_health> : Inport
  Add : Sum
  Cast To Single : DataTypeConversion  OutDataTypeStr=single  SaturateOnIntegerOverflow=off  RndMeth=Floor
  Constant : Constant  Value=-0.5
  Gain : Gain  Gain=2
  Subsystem : Subsystem
  inceptor_health_filtered : Outport
  wires:
  Subsystem/1(incept_health_filter) -> inceptor_health_filtered/1
  <inceptor_health>/1 -> Cast To Single/1
  Cast To Single/1 -> Add/1
  Constant/1 -> Add/2
  Gain/1 -> Subsystem/1(<incept_health_raw>)
  Add/1 -> Gain/1

== system malt_test_angle/determine arm and mode selection/Failsafe_management/Radio failsafe/Subsystem/Subsystem ==
  <incept_health_raw> : Inport
  Abs1 : Abs  SaturateOnIntegerOverflow=off
  Compare To Constant : simulink/Logic and Bit Operations/Compare To Constant  relop=>=  const=0.98  OutDataTypeStr=boolean
  e_stop counter : Subsystem
  incept_health_filter : Outport
  wires:
  Compare To Constant/1 -> e_stop counter/Enable
  Abs1/1 -> Compare To Constant/1
  <incept_health_raw>/1 -> e_stop counter/1(motor_e_stop_raw), Abs1/1
  e_stop counter/1(e_stop_filtered) -> incept_health_filter/1

== system malt_test_angle/determine arm and mode selection/Failsafe_management/Radio failsafe/Subsystem/Subsystem/e_stop counter ==
  note: This is to ensure e_stop event is not triggered unless e_stop command is sent for more than 0.3 s to prevent false trigger
  motor_e_stop_raw : Inport
  Enable : EnablePort  StatesWhenEnabling=reset
  Compare To Constant : simulink/Logic and Bit Operations/Compare To Constant  relop=>=  const=0.5  OutDataTypeStr=boolean
  Discrete-Time Integrator : DiscreteIntegrator  SampleTime=0.01  LimitOutput=on  UpperSaturationLimit=1  LowerSaturationLimit=0  ICPrevOutput=DiscIntNeverNeededParam  ICPrevScaledInput=DiscIntNeverNeededParam
  Gain : Gain  Gain=2
  e_stop_filtered : Outport
  wires:
  Compare To Constant/1 -> e_stop_filtered/1
  Discrete-Time Integrator/1 -> Compare To Constant/1
  Gain/1 -> Discrete-Time Integrator/1
  motor_e_stop_raw/1 -> Gain/1

== matlab function malt_test_angle/ANGLE CONTROLLER1/Roll Controller/roll_D_DLPF/MATLAB Function ==
  data: prev_val input; raw_val input; filtered_val output; freq_cut input
function filtered_val = IIR_filt( prev_val,raw_val, freq_cut)
    fc = freq_cut/100;
    b = 2 - cos(2 * pi * fc) - sqrt((2 - cos(2 * pi * fc))^2 - 1);
    a = 1 - b;
    filtered_val = a * raw_val + b * prev_val;

== matlab function malt_test_angle/Stab_input_conversion/remap from min_spin to max/remap1 ==
  data: raw_in input; norm_out output; in_min input; in_max input; out_min input; out_max input
function norm_out = remap(raw_in,in_min,in_max,out_min,out_max)
norm_out = (raw_in - in_min) * (out_max - out_min)/(in_max-in_min) + out_min;

== matlab function malt_test_angle/cmd to raw pwm1/motor_PWM_denormalize/remap ==
  data: norm_in input; raw_out output; in_min input; in_max input; out_min input; out_max input
function raw_out = remap(norm_in,in_min,in_max,out_min,out_max)
raw_out = (norm_in - in_min) * (out_max - out_min)/(in_max-in_min) + out_min;

== matlab function malt_test_angle/command selection/yaw_norm_deadband/remap_with_deadband ==
  data: raw_in input; norm_out output; in_min input; in_max input; out_min input; out_max input; deadband input
function norm_out = remap_deadband(raw_in, in_min, in_max, out_min, out_max, deadband)
in_avg = (in_min + in_max) / 2;
out_avg = (out_min + out_max) / 2;

in_deadband_range = (in_max - in_min) * deadband / 2;
in_deadband_low = in_avg - in_deadband_range;
in_deadband_hi = in_avg + in_deadband_range;

if raw_in < in_deadband_low
    norm_out = (raw_in - in_deadband_low) .* (out_max - out_avg)./(in_deadband_low - in_min) + out_avg;
elseif raw_in > in_deadband_low && raw_in < in_deadband_hi
    norm_out = out_avg;
else
    norm_out = (raw_in - in_deadband_hi) .* (out_max - out_avg)./(in_max - in_deadband_hi) + out_avg;
end

== matlab function malt_test_angle/ANGLE CONTROLLER1/Pitch Controller/Pitch_D_DLPF/MATLAB Function ==
  data: prev_val input; raw_val input; filtered_val output; freq_cut input
function filtered_val = IIR_filt( prev_val,raw_val, freq_cut)
    fc = freq_cut/100;
    b = 2 - cos(2 * pi * fc) - sqrt((2 - cos(2 * pi * fc))^2 - 1);
    a = 1 - b;
    filtered_val = a * raw_val + b * prev_val;

== matlab function malt_test_angle/ANGLE CONTROLLER1/Yaw Rate Controller/yaw_D_DLPF/MATLAB Function ==
  data: prev_val input; raw_val input; filtered_val output; freq_cut input
function filtered_val = IIR_filt( prev_val,raw_val, freq_cut)
    fc = freq_cut/100;
    b = 2 - cos(2 * pi * fc) - sqrt((2 - cos(2 * pi * fc))^2 - 1);
    a = 1 - b;
    filtered_val = a * raw_val + b * prev_val;

== matlab function malt_test_angle/command selection/throttle_norm/remap ==
  data: raw_in input; norm_out output; in_min input; in_max input; out_min input; out_max input
function norm_out = remap(raw_in,in_min,in_max,out_min,out_max)
norm_out = (raw_in - in_min) * (out_max - out_min)/(in_max-in_min) + out_min;

== matlab function malt_test_angle/Stab_input_conversion1/pitch_norm_deadband/remap_with_deadband ==
  data: raw_in input; norm_out output; in_min input; in_max input; out_min input; out_max input; deadband input
function norm_out = remap_deadband(raw_in, in_min, in_max, out_min, out_max, deadband)
in_avg = (in_min + in_max) / 2;
out_avg = (out_min + out_max) / 2;

in_deadband_range = (in_max - in_min) * deadband / 2;
in_deadband_low = in_avg - in_deadband_range;
in_deadband_hi = in_avg + in_deadband_range;

if raw_in < in_deadband_low
    norm_out = (raw_in - in_deadband_low) .* (out_max - out_avg)./(in_deadband_low - in_min) + out_avg;
elseif raw_in > in_deadband_low && raw_in < in_deadband_hi
    norm_out = out_avg;
else
    norm_out = (raw_in - in_deadband_hi) .* (out_max - out_avg)./(in_max - in_deadband_hi) + out_avg;
end

== matlab function malt_test_angle/command selection/roll_norm_deadband/remap_with_deadband ==
  data: raw_in input; norm_out output; in_min input; in_max input; out_min input; out_max input; deadband input
function norm_out = remap_deadband(raw_in, in_min, in_max, out_min, out_max, deadband)
in_avg = (in_min + in_max) / 2;
out_avg = (out_min + out_max) / 2;

in_deadband_range = (in_max - in_min) * deadband / 2;
in_deadband_low = in_avg - in_deadband_range;
in_deadband_hi = in_avg + in_deadband_range;

if raw_in < in_deadband_low
    norm_out = (raw_in - in_deadband_low) .* (out_max - out_avg)./(in_deadband_low - in_min) + out_avg;
elseif raw_in > in_deadband_low && raw_in < in_deadband_hi
    norm_out = out_avg;
else
    norm_out = (raw_in - in_deadband_hi) .* (out_max - out_avg)./(in_max - in_deadband_hi) + out_avg;
end

== matlab function malt_test_angle/command selection/pitch_norm_deadband/remap_with_deadband ==
  data: raw_in input; norm_out output; in_min input; in_max input; out_min input; out_max input; deadband input
function norm_out = remap_deadband(raw_in, in_min, in_max, out_min, out_max, deadband)
in_avg = (in_min + in_max) / 2;
out_avg = (out_min + out_max) / 2;

in_deadband_range = (in_max - in_min) * deadband / 2;
in_deadband_low = in_avg - in_deadband_range;
in_deadband_hi = in_avg + in_deadband_range;

if raw_in < in_deadband_low
    norm_out = (raw_in - in_deadband_low) .* (out_max - out_avg)./(in_deadband_low - in_min) + out_avg;
elseif raw_in > in_deadband_low && raw_in < in_deadband_hi
    norm_out = out_avg;
else
    norm_out = (raw_in - in_deadband_hi) .* (out_max - out_avg)./(in_max - in_deadband_hi) + out_avg;
end

== matlab function malt_test_angle/command selection/e_stop_norm/remap ==
  data: raw_in input; norm_out output; in_min input; in_max input; out_min input; out_max input
function norm_out = remap(raw_in,in_min,in_max,out_min,out_max)
norm_out = (raw_in - in_min) * (out_max - out_min)/(in_max-in_min) + out_min;

== matlab function malt_test_angle/command selection/mode_norm/remap ==
  data: raw_in input; norm_out output; in_min input; in_max input; out_min input; out_max input
function norm_out = remap(raw_in,in_min,in_max,out_min,out_max)
norm_out = (raw_in - in_min) * (out_max - out_min)/(in_max-in_min) + out_min;

== matlab function malt_test_angle/POS_HOLD CONTROLLER/Vertical speed controller/MATLAB Function ==
  data: prev_val input; raw_val input; filtered_val output; freq_cut input
function filtered_val = IIR_filt( prev_val,raw_val, freq_cut)
    fc = freq_cut/100;
    b = 2 - cos(2 * pi * fc) - sqrt((2 - cos(2 * pi * fc))^2 - 1);
    a = 1 - b;
    filtered_val = a * raw_val + b * prev_val;
